simulink model "mrm_controller"  (R2025b)
settings: Solver=VariableStepAuto  StartTime=0.0  StopTime=10.0  RelTol=1e-3
settings Model: Creator=hubertm  LastModifiedBy=hubertm

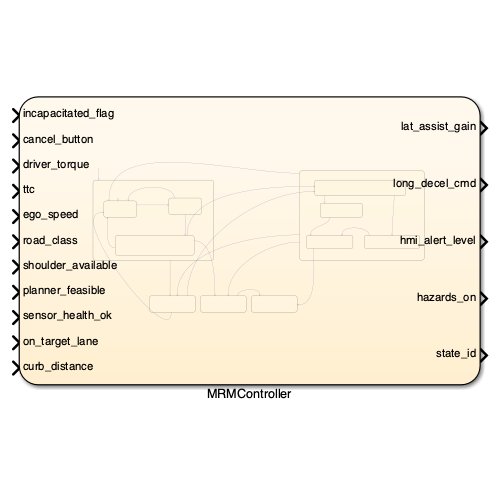
[thumbnail: Simulink's stored preview of the top-level diagram]
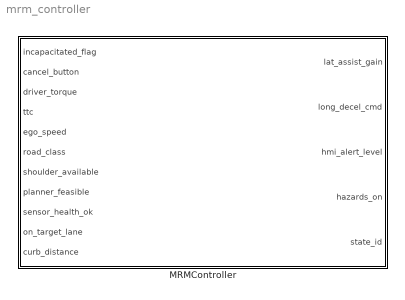
== system mrm_controller ==
  MRMController : Stateflow chart  TreatAsAtomicUnit=on

== stateflow chart mrm_controller/MRMController ==
  state MRM
    state MRM_Plan
      entry:
      lat_assist_gain = 1.0;
      long_decel_cmd  = DECEL_MRM;
      hazards_on      = true;
      state_id        = uint8(4);
    state MRM_HighwayPullOver
      entry: state_id = uint8(5);
    state MRM_Stopping
      entry:
      long_decel_cmd = DECEL_MRM;
      state_id       = uint8(7);
    state MRM_UrbanPullOver
      entry: state_id = uint8(6);
    MRM_Plan -> MRM_HighwayPullOver [order 1] : [(road_class==uint8(0)||road_class==uint8(1)) && shoulder_available && planner_feasible]
    MRM_Plan -> MRM_UrbanPullOver [order 2] : [(road_class==uint8(2)||road_class==uint8(3)) && planner_feasible]
    MRM_HighwayPullOver -> MRM_Stopping : [on_target_lane]
    MRM_UrbanPullOver -> MRM_Stopping : [on_target_lane && curb_distance < 0.5]
  state NOMINAL
    state AttentionWarning
      entry:
      hmi_alert_level = uint8(1);
      state_id        = uint8(2);
    state DriverFullControl
      entry:
      lat_assist_gain = 0;
      long_decel_cmd  = 0;
      hmi_alert_level = uint8(0);
      hazards_on      = false;
      state_id        = uint8(1);
    state TransitionDemand
      entry:
      hmi_alert_level = uint8(3);
      long_decel_cmd  = DECEL_MRM * 0.5;
      state_id        = uint8(3);
      during:
      lat_assist_gain = 1.0/(1.0 + exp(-1.0*(temporalCount(sec) - TD_DURATION/2)));
    AttentionWarning -> DriverFullControl [order 1] : [~incapacitated_flag || cancel_button]
    (default) -> DriverFullControl
    DriverFullControl -> AttentionWarning : [incapacitated_flag]
    AttentionWarning -> TransitionDemand [order 2] : [after(AW_DURATION,sec) && incapacitated_flag]
    TransitionDemand -> DriverFullControl [order 1] : [abs(driver_torque) > TORQUE_OVERRIDE || cancel_button]
  state EM
    entry:
    long_decel_cmd  = DECEL_EM;
    hmi_alert_level = uint8(3);
    hazards_on      = true;
    state_id        = uint8(8);
  state Fault
    entry:
    long_decel_cmd = DECEL_MRM;
    hazards_on     = true;
    state_id       = uint8(9);
  state Stopped
    entry:
    long_decel_cmd = 0;
    hazards_on     = true;
    state_id       = uint8(10);
  MRM -> DriverFullControl [order 1] : [cancel_button]
  (default) -> NOMINAL
  TransitionDemand -> MRM_Plan [order 2] : [after(TD_DURATION,sec) && incapacitated_flag]
  EM -> MRM_Plan [order 1] : [ttc > TTC_EM*2 &&  incapacitated_flag]
  EM -> DriverFullControl [order 2] : [ttc > TTC_EM*2 && ~incapacitated_flag]
  MRM -> EM [order 2] : [ttc < TTC_EM]
  TransitionDemand -> Fault [order 3] : [~sensor_health_ok]
  MRM -> Fault [order 3] : [~sensor_health_ok || ~planner_feasible]
  MRM_Stopping -> Stopped : [ego_speed < 0.1]
  NOMINAL -> EM : [ttc < TTC_EM]
  Fault -> Stopped : [ego_speed < 0.1]
  data: incapacitated_flag input boolean; cancel_button input boolean; driver_torque input double; ttc input double; ego_speed input double; road_class input uint8; shoulder_available input boolean; planner_feasible input boolean; sensor_health_ok input boolean; on_target_lane input boolean; curb_distance input double; lat_assist_gain output double; long_decel_cmd output double; hmi_alert_level output uint8; hazards_on output boolean; state_id output uint8; TD_DURATION constant double =10; AW_DURATION constant double =4; TTC_EM constant double =2.0; DECEL_EM constant double =5.0; DECEL_MRM constant double =2.5; TORQUE_OVERRIDE constant double =3.0
